simulink model "DvrSimKeybdGD_cs_old"  (R2016a)
settings: Solver=ode5  SolverMode=SingleTasking  StartTime=0.0  StopTime=inf  FixedStep=1/1000  RelTol=1e-3
PreLoadFcn:
  | mbxruntime.callbacks.PreLoadFcn(bdroot);
PostLoadFcn:
  | mbxruntime.callbacks.PostLoadFcn(bdroot);
InitFcn:
  | mbxruntime.callbacks.InitFcn(bdroot);
StartFcn:
  | mbxruntime.callbacks.StartFcn(bdroot);
StopFcn:
  | mbxruntime.callbacks.StopFcn(bdroot);
model workspace (MAT data in the model file):
  mbox_table : struct (value not decoded)
  model_closed = 0
  sim_status = 0
undefined symbols (not defined in the file or in its folder): BMotor1, BMotor2, BrkDelayTime, DControlB, Delay1, Delay2, DiscIntNeverNeededParam, IControlB, JMotor1, JMotor2, PControlB, PreScanCarSimLoadFcn, ratioGearF, ratioGearR, TorqDelayTime, Tstep
undefined symbols (not defined in the file): SteeringColumn, SteeringWheel, WheelL0, WheelL1, WheelR0, WheelR1
libraries: PreScanSimulinkLibrary x35, simulink_extras x26, simulink x26, MyLib x3, Solver_SF x2, pil_lib x1, PreScanUsefulBlocks x1
(part 3 of 12)

== system DvrSimKeybdGD_cs_old/Audi_A8_Sedan_1/Trajectories ==
  Constant1 : Constant  Value=30
  Constant2 : Constant  Value=50
  Discrete-Time Integrator : DiscreteIntegrator  ExternalReset=rising  InitialConditionSource=external  SampleTime=1/20  ICPrevOutput=DiscIntNeverNeededParam  ICPrevScaledInput=DiscIntNeverNeededParam
  ElapsedTrack1 : Subsystem  Tag=ElapsedTrack  mask(PreScan Demux Block:){Filename='Trajectory_2_Path.mat', InitRoll=0, InitPitch=0}
      mask prompts: Filename "Name path-file"; InitRoll "Initial Roll angle (deg):"; InitPitch "Initial Pitch angle (deg):"
      mask init:
      | route=load(['trajectories/',Filename]);
      | 
      | s=route.path(1,:);
      | x=route.path(2,:);
      | y=route.path(3,:);
      | z=route.path(4,:);
      | roll=route.path(5,:);
      | pitch=route.path(6,:);
      | yaw=route.path(7,:);
      settings: DeleteFcn=PreScanBlockDeleteFcn;
  End of Track is reached : Subsystem  Tag=ElapsedTrack  mask(PreScan Demux Block:){Filename='Trajectory_2_Path.mat'}
      mask prompts: Filename "Name path-file"
      mask init:
      | route=load(['trajectories/',Filename]);
      | 
      | s=route.path(1,:);
      | x=route.path(2,:);
      | y=route.path(3,:);
      | yaw=route.path(4,:);
      settings: DeleteFcn=PreScanBlockDeleteFcn;
  Gain : Gain  Gain=1/3.6
  Integrator1 : DiscreteIntegrator  Tag=TrajIntegrator  InitialConditionSetting=State (most efficient)  SampleTime=50/1000  ICPrevOutput=DiscIntNeverNeededParam  ICPrevScaledInput=DiscIntNeverNeededParam
  Memory1 : Memory
  Product : Product  RndMeth=Zero
  Selector1 : Constant  Tag=TrajSubSelector  Value=2
  Step : Step  Before=1  After=0  SampleTime=0
  Terminator_1 : Terminator
  Traj2State1 : Subsystem  Tag=Traj2State  mask(PreScan Demux Block:){}
      settings: DeleteFcn=PreScanBlockDeleteFcn;
  TrajCoGOffset : Subsystem  Tag=TrajCoGOffset  mask(Trajectory CoG Offset block){CoGOffsetZ=0.55, InitRoll=0, InitPitch=0}
      mask prompts: CoGOffsetZ "Z-component of CoG Offset [m]:"; InitRoll "Initial Roll angle [deg]:"; InitPitch "Initial Pitch angle [deg]:"
      mask help: A trajectory follows the surface of the road. However the position of a actor is based on the actor's Center of Gravity, which is typically above the road. This block converts from the trajectory along the road surface to the trajectory of the actor's CoG by realigning the z-component of the CoG offset to be normal to the road.
      settings: DeleteFcn=PreScanBlockDeleteFcn;
  TrajSwitch1 : MultiPortSwitch  Tag=TrajSubSwitch  Inputs=2
  Trajectory_2 : Subsystem  Tag=Trajectory  mask(PreScan Source Block: Trajectory){FileName='Trajectory_2.mat', TimeStep=50/1000}
      mask prompts: TimeStep "Time Step [s]"
      mask help:
      | The Trajectory block contains the trajectories defined in the PreScan Experiment Editor. The output of the trajectory block is the (vehicle) State.
      |
      | For more information, please click Help.
      mask init:
      | EXPROOT=pwd;  % TODO better construction for locating base experiment
      | 
      | trajfilename = fullfile(EXPROOT,'Trajectories',FileName);
      | load(trajfilename);
      | trajectory=trajectory';
      | 
      | traj.time=trajectory(:,1);%[];
      | traj.signals.values=trajectory(:,2:19);
      | traj.dimensions=18;
      | traj.label='';
      | 
      | SampleTime=traj.time(2)-traj.time(1);
      settings: DeleteFcn=PreScanBlockDeleteFcn;
      mask Help: eval('openHelp(312)')
      mask Display: fprintf(FileName)
  Trajectory_2_Offset : Constant  Tag=TrajectoryOffset  Value="[0  0  0  0  0  0]"
  Velocity1 : Constant  Tag=TrajVelocity  Value=15
  State : Outport  Tag=TrajOutport
  wires:
  Constant2/1 -> Product/1
  Product/1 -> Discrete-Time Integrator/3
  Discrete-Time Integrator/1 -> ElapsedTrack1/2(s), Memory1/1
  Memory1/1 -> End of Track is reached/1(s)
  End of Track is reached/1(end_reached) -> Discrete-Time Integrator/2
  Gain/1 -> Discrete-Time Integrator/1
  Constant1/1 -> Gain/1
  Step/1 -> Product/2
  Integrator1/1 -> Terminator_1/1
  Trajectory_2/1(trajectory) -> Traj2State1/1(Traj Org)
  Trajectory_2_Offset/1 -> Traj2State1/2(Offset), ElapsedTrack1/1(Offset)
  Velocity1/1 -> Integrator1/1
  Selector1/1 -> TrajSwitch1/1
  Traj2State1/1(state) -> TrajSwitch1/2
  ElapsedTrack1/1(state) -> TrajSwitch1/3
  TrajCoGOffset/1(State Out) -> State/1
  TrajSwitch1/1 -> TrajCoGOffset/1(State In)

== system DvrSimKeybdGD_cs_old/BMW_X5_SUV_1/SELF_Demux ==
  SELF : Inport  OutDataTypeStr=Bus: PRESCAN_SELFSENSORDATA
  Bus Selector : BusSelector  OutputSignals=PositionX,PositionY,PositionZ,OrientationRoll,OrientationPitch,OrientationYaw,Velocity,Yaw_rate,Lat,Long,Alt
  Demux2 : Demux  Outputs=3
  Gain : Gain  Gain=180/pi
  Gain1 : Gain  Gain=180/pi
  Vector Concatenate1 : Concatenate  NumInputs=3
  compas converter : Subsystem
  x [m] : Outport
  y [m] : Outport  Port=2
  z [m] : Outport  Port=3
  rotx [deg] : Outport  Port=4
  roty [deg] : Outport  Port=5
  rotz [deg] : Outport  Port=6
  GPS lat [deg] : Outport  Port=7
  GPS long [deg] : Outport  Port=8
  GPS alt [m] : Outport  Port=9
  velocity [m/s] : Outport  Port=10
  heading [deg] : Outport  Port=11
  yaw rate [deg/s] : Outport  Port=12
  wires:
  Bus Selector/11 -> GPS alt [m]/1  "<Alt>"
  Bus Selector/10 -> GPS long [deg]/1  "<Long>"
  Bus Selector/9 -> GPS lat [deg]/1  "<Lat>"
  Bus Selector/8 -> Gain1/1  "<Yaw_rate>"
  Bus Selector/7 -> velocity [m/s]/1  "<Velocity>"
  Bus Selector/6 -> compas converter/1(rotz [rad]), Vector Concatenate1/3  "<OrientationYaw>"
  Bus Selector/5 -> Vector Concatenate1/2  "<OrientationPitch>"
  Bus Selector/4 -> Vector Concatenate1/1  "<OrientationRoll>"
  Vector Concatenate1/1 -> Gain/1
  Bus Selector/3 -> z [m]/1  "<PositionZ>"
  Bus Selector/2 -> y [m]/1  "<PositionY>"
  Bus Selector/1 -> x [m]/1  "<PositionX>"
  SELF/1 -> Bus Selector/1
  Gain/1 -> Demux2/1
  Demux2/1 -> rotx [deg]/1
  Demux2/2 -> roty [deg]/1
  Demux2/3 -> rotz [deg]/1
  compas converter/1(heading [deg]) -> heading [deg]/1
  Gain1/1 -> yaw rate [deg/s]/1

== system DvrSimKeybdGD_cs_old/BMW_X5_SUV_1/STATE_BMW_X5_SUV_1 ==
  State : Inport  SampleTime=TimeStep
  Bus Creator : BusCreator  Inputs=15  OutDataTypeStr=Bus: PRESCAN_STATEACTUATORDATA  NonVirtualBus=on
  Demux : Demux  Outputs=15
  iniBODYAngles wrtVEH [rad] : Constant  Value=[Roll0 Pitch0 0]  SampleTime=TimeStep
  iniVEHAngles wrtGLOB [rad] : Constant  Value=[0 0 Yaw0]  SampleTime=TimeStep
  iniVEHposition wrtGLOB [m] : Constant  Value=[x0 y0 z0]  SampleTime=TimeStep
  state2FullState : PreScanSimulinkLibrary/state2FullState  SystemSampleTime=-1
  StateBus : Outport  OutDataTypeStr=Bus: PRESCAN_STATEACTUATORDATA
  wires:
  Bus Creator/1 -> StateBus/1
  State/1 -> state2FullState/1
  state2FullState/1 -> Demux/1
  iniVEHposition wrtGLOB [m]/1 -> state2FullState/2
  iniBODYAngles wrtVEH [rad]/1 -> state2FullState/3
  iniVEHAngles wrtGLOB [rad]/1 -> state2FullState/4
  Demux/1 -> Bus Creator/1  "PositionX"
  Demux/2 -> Bus Creator/2  "PositionY"
  Demux/3 -> Bus Creator/3  "PositionZ"
  Demux/4 -> Bus Creator/4  "VelocityX"
  Demux/5 -> Bus Creator/5  "VelocityY"
  Demux/6 -> Bus Creator/6  "VelocityZ"
  Demux/7 -> Bus Creator/7  "AccelerationX"
  Demux/8 -> Bus Creator/8  "AccelerationY"
  Demux/9 -> Bus Creator/9  "AccelerationZ"
  Demux/10 -> Bus Creator/10  "OrientationRoll"
  Demux/11 -> Bus Creator/11  "OrientationPitch"
  Demux/12 -> Bus Creator/12  "OrientationYaw"
  Demux/13 -> Bus Creator/13  "AngularVelocityRoll"
  Demux/14 -> Bus Creator/14  "AngularVelocityPitch"
  Demux/15 -> Bus Creator/15  "AngularVelocityYaw"

== system DvrSimKeybdGD_cs_old/BMW_X5_SUV_1/Trajectories ==
  Constant1 : Constant  Value=30
  Constant2 : Constant  Value=50
  Discrete-Time Integrator : DiscreteIntegrator  ExternalReset=rising  InitialConditionSource=external  SampleTime=1/20  ICPrevOutput=DiscIntNeverNeededParam  ICPrevScaledInput=DiscIntNeverNeededParam
  ElapsedTrack1 : Subsystem  Tag=ElapsedTrack  mask(PreScan Demux Block:){Filename='Trajectory_4_Path.mat', InitRoll=0, InitPitch=0}
      mask prompts: Filename "Name path-file"; InitRoll "Initial Roll angle (deg):"; InitPitch "Initial Pitch angle (deg):"
      mask init:
      | route=load(['trajectories/',Filename]);
      | 
      | s=route.path(1,:);
      | x=route.path(2,:);
      | y=route.path(3,:);
      | z=route.path(4,:);
      | roll=route.path(5,:);
      | pitch=route.path(6,:);
      | yaw=route.path(7,:);
      settings: DeleteFcn=PreScanBlockDeleteFcn;
  End of Track is reached : Subsystem  Tag=ElapsedTrack  mask(PreScan Demux Block:){Filename='Trajectory_4_Path.mat'}
      mask prompts: Filename "Name path-file"
      mask init:
      | route=load(['trajectories/',Filename]);
      | 
      | s=route.path(1,:);
      | x=route.path(2,:);
      | y=route.path(3,:);
      | yaw=route.path(4,:);
      settings: DeleteFcn=PreScanBlockDeleteFcn;
  Gain : Gain  Gain=1/3.6
  Integrator1 : DiscreteIntegrator  Tag=TrajIntegrator  InitialConditionSetting=State (most efficient)  SampleTime=50/1000  ICPrevOutput=DiscIntNeverNeededParam  ICPrevScaledInput=DiscIntNeverNeededParam
  Memory1 : Memory
  Product : Product  RndMeth=Zero
  Selector1 : Constant  Tag=TrajSubSelector  Value=2
  Step : Step  Before=1  After=0  SampleTime=0
  Terminator_1 : Terminator
  Traj2State1 : Subsystem  Tag=Traj2State  mask(PreScan Demux Block:){}
      settings: DeleteFcn=PreScanBlockDeleteFcn;
  TrajCoGOffset : Subsystem  Tag=TrajCoGOffset  mask(Trajectory CoG Offset block){CoGOffsetZ=0.69, InitRoll=0, InitPitch=0}
      mask prompts: CoGOffsetZ "Z-component of CoG Offset [m]:"; InitRoll "Initial Roll angle [deg]:"; InitPitch "Initial Pitch angle [deg]:"
      mask help: A trajectory follows the surface of the road. However the position of a actor is based on the actor's Center of Gravity, which is typically above the road. This block converts from the trajectory along the road surface to the trajectory of the actor's CoG by realigning the z-component of the CoG offset to be normal to the road.
      settings: DeleteFcn=PreScanBlockDeleteFcn;
  TrajSwitch1 : MultiPortSwitch  Tag=TrajSubSwitch  Inputs=2
  Trajectory_4 : Subsystem  Tag=Trajectory  mask(PreScan Source Block: Trajectory){FileName='Trajectory_4.mat', TimeStep=50/1000}
      mask prompts: TimeStep "Time Step [s]"
      mask help:
      | The Trajectory block contains the trajectories defined in the PreScan Experiment Editor. The output of the trajectory block is the (vehicle) State.
      |
      | For more information, please click Help.
      mask init: same as DvrSimKeybdGD_cs_old/Audi_A8_Sedan_1/Trajectories/Trajectory_2
      settings: DeleteFcn=PreScanBlockDeleteFcn;
      mask Help: eval('openHelp(312)')
      mask Display: fprintf(FileName)
  Trajectory_4_Offset : Constant  Tag=TrajectoryOffset  Value="[0  0  0  0  0  0]"
  Velocity1 : Constant  Tag=TrajVelocity  Value=15
  State : Outport  Tag=TrajOutport
  wires:
  Constant2/1 -> Product/1
  Product/1 -> Discrete-Time Integrator/3
  Discrete-Time Integrator/1 -> ElapsedTrack1/2(s), Memory1/1
  Memory1/1 -> End of Track is reached/1(s)
  End of Track is reached/1(end_reached) -> Discrete-Time Integrator/2
  Gain/1 -> Discrete-Time Integrator/1
  Constant1/1 -> Gain/1
  Step/1 -> Product/2
  Integrator1/1 -> Terminator_1/1
  Trajectory_4/1(trajectory) -> Traj2State1/1(Traj Org)
  Trajectory_4_Offset/1 -> Traj2State1/2(Offset), ElapsedTrack1/1(Offset)
  Velocity1/1 -> Integrator1/1
  Selector1/1 -> TrajSwitch1/1
  Traj2State1/1(state) -> TrajSwitch1/2
  ElapsedTrack1/1(state) -> TrajSwitch1/3
  TrajCoGOffset/1(State Out) -> State/1
  TrajSwitch1/1 -> TrajCoGOffset/1(State In)

== system DvrSimKeybdGD_cs_old/BMW_Z3_Convertible_1/SELF_Demux ==
  SELF : Inport  OutDataTypeStr=Bus: PRESCAN_SELFSENSORDATA
  Bus Selector : BusSelector  OutputSignals=PositionX,PositionY,PositionZ,OrientationRoll,OrientationPitch,OrientationYaw,Velocity,Yaw_rate,Lat,Long,Alt
  Demux2 : Demux  Outputs=3
  Gain : Gain  Gain=180/pi
  Gain1 : Gain  Gain=180/pi
  Vector Concatenate1 : Concatenate  NumInputs=3
  compas converter : Subsystem
  x [m] : Outport
  y [m] : Outport  Port=2
  z [m] : Outport  Port=3
  rotx [deg] : Outport  Port=4
  roty [deg] : Outport  Port=5
  rotz [deg] : Outport  Port=6
  GPS lat [deg] : Outport  Port=7
  GPS long [deg] : Outport  Port=8
  GPS alt [m] : Outport  Port=9
  velocity [m/s] : Outport  Port=10
  heading [deg] : Outport  Port=11
  yaw rate [deg/s] : Outport  Port=12
  wires:
  Bus Selector/11 -> GPS alt [m]/1  "<Alt>"
  Bus Selector/10 -> GPS long [deg]/1  "<Long>"
  Bus Selector/9 -> GPS lat [deg]/1  "<Lat>"
  Bus Selector/8 -> Gain1/1  "<Yaw_rate>"
  Bus Selector/7 -> velocity [m/s]/1  "<Velocity>"
  Bus Selector/6 -> compas converter/1(rotz [rad]), Vector Concatenate1/3  "<OrientationYaw>"
  Bus Selector/5 -> Vector Concatenate1/2  "<OrientationPitch>"
  Bus Selector/4 -> Vector Concatenate1/1  "<OrientationRoll>"
  Vector Concatenate1/1 -> Gain/1
  Bus Selector/3 -> z [m]/1  "<PositionZ>"
  Bus Selector/2 -> y [m]/1  "<PositionY>"
  Bus Selector/1 -> x [m]/1  "<PositionX>"
  SELF/1 -> Bus Selector/1
  Gain/1 -> Demux2/1
  Demux2/1 -> rotx [deg]/1
  Demux2/2 -> roty [deg]/1
  Demux2/3 -> rotz [deg]/1
  compas converter/1(heading [deg]) -> heading [deg]/1
  Gain1/1 -> yaw rate [deg/s]/1

== system DvrSimKeybdGD_cs_old/BMW_Z3_Convertible_1/STATE_BMW_Z3_Convertible_1 ==
  State : Inport  SampleTime=TimeStep
  Bus Creator : BusCreator  Inputs=15  OutDataTypeStr=Bus: PRESCAN_STATEACTUATORDATA  NonVirtualBus=on
  Demux : Demux  Outputs=15
  iniBODYAngles wrtVEH [rad] : Constant  Value=[Roll0 Pitch0 0]  SampleTime=TimeStep
  iniVEHAngles wrtGLOB [rad] : Constant  Value=[0 0 Yaw0]  SampleTime=TimeStep
  iniVEHposition wrtGLOB [m] : Constant  Value=[x0 y0 z0]  SampleTime=TimeStep
  state2FullState : PreScanSimulinkLibrary/state2FullState  SystemSampleTime=-1
  StateBus : Outport  OutDataTypeStr=Bus: PRESCAN_STATEACTUATORDATA
  wires:
  Bus Creator/1 -> StateBus/1
  State/1 -> state2FullState/1
  state2FullState/1 -> Demux/1
  iniVEHposition wrtGLOB [m]/1 -> state2FullState/2
  iniBODYAngles wrtVEH [rad]/1 -> state2FullState/3
  iniVEHAngles wrtGLOB [rad]/1 -> state2FullState/4
  Demux/1 -> Bus Creator/1  "PositionX"
  Demux/2 -> Bus Creator/2  "PositionY"
  Demux/3 -> Bus Creator/3  "PositionZ"
  Demux/4 -> Bus Creator/4  "VelocityX"
  Demux/5 -> Bus Creator/5  "VelocityY"
  Demux/6 -> Bus Creator/6  "VelocityZ"
  Demux/7 -> Bus Creator/7  "AccelerationX"
  Demux/8 -> Bus Creator/8  "AccelerationY"
  Demux/9 -> Bus Creator/9  "AccelerationZ"
  Demux/10 -> Bus Creator/10  "OrientationRoll"
  Demux/11 -> Bus Creator/11  "OrientationPitch"
  Demux/12 -> Bus Creator/12  "OrientationYaw"
  Demux/13 -> Bus Creator/13  "AngularVelocityRoll"
  Demux/14 -> Bus Creator/14  "AngularVelocityPitch"
  Demux/15 -> Bus Creator/15  "AngularVelocityYaw"

== system DvrSimKeybdGD_cs_old/BMW_Z3_Convertible_1/Trajectories ==
  Constant1 : Constant  Value=60
  Constant2 : Constant  Value=200
  Discrete-Time Integrator : DiscreteIntegrator  ExternalReset=rising  InitialConditionSource=external  SampleTime=1/20  ICPrevOutput=DiscIntNeverNeededParam  ICPrevScaledInput=DiscIntNeverNeededParam
  ElapsedTrack1 : Subsystem  Tag=ElapsedTrack  mask(PreScan Demux Block:){Filename='Trajectory_1_Path.mat', InitRoll=0, InitPitch=0}
      mask prompts: Filename "Name path-file"; InitRoll "Initial Roll angle (deg):"; InitPitch "Initial Pitch angle (deg):"
      mask init:
      | route=load(['trajectories/',Filename]);
      | 
      | s=route.path(1,:);
      | x=route.path(2,:);
      | y=route.path(3,:);
      | z=route.path(4,:);
      | roll=route.path(5,:);
      | pitch=route.path(6,:);
      | yaw=route.path(7,:);
      settings: DeleteFcn=PreScanBlockDeleteFcn;
  End of Track is reached : Subsystem  Tag=ElapsedTrack  mask(PreScan Demux Block:){Filename='Trajectory_1_Path.mat'}
      mask prompts: Filename "Name path-file"
      mask init:
      | route=load(['trajectories/',Filename]);
      | 
      | s=route.path(1,:);
      | x=route.path(2,:);
      | y=route.path(3,:);
      | yaw=route.path(4,:);
      settings: DeleteFcn=PreScanBlockDeleteFcn;
  Gain : Gain  Gain=1/3.6
  Integrator1 : DiscreteIntegrator  Tag=TrajIntegrator  InitialConditionSetting=State (most efficient)  SampleTime=50/1000  ICPrevOutput=DiscIntNeverNeededParam  ICPrevScaledInput=DiscIntNeverNeededParam
  Memory1 : Memory
  Product : Product  RndMeth=Zero
  Selector1 : Constant  Tag=TrajSubSelector  Value=2
  Step : Step  Before=1  After=0  SampleTime=0
  Terminator_1 : Terminator
  Traj2State1 : Subsystem  Tag=Traj2State  mask(PreScan Demux Block:){}
      settings: DeleteFcn=PreScanBlockDeleteFcn;
  TrajCoGOffset : Subsystem  Tag=TrajCoGOffset  mask(Trajectory CoG Offset block){CoGOffsetZ=0.4784, InitRoll=0, InitPitch=0}
      mask prompts: CoGOffsetZ "Z-component of CoG Offset [m]:"; InitRoll "Initial Roll angle [deg]:"; InitPitch "Initial Pitch angle [deg]:"
      mask help: A trajectory follows the surface of the road. However the position of a actor is based on the actor's Center of Gravity, which is typically above the road. This block converts from the trajectory along the road surface to the trajectory of the actor's CoG by realigning the z-component of the CoG offset to be normal to the road.
      settings: DeleteFcn=PreScanBlockDeleteFcn;
  TrajSwitch1 : MultiPortSwitch  Tag=TrajSubSwitch  Inputs=2
  Trajectory_1 : Subsystem  Tag=Trajectory  mask(PreScan Source Block: Trajectory){FileName='Trajectory_1.mat', TimeStep=50/1000}
      mask prompts: TimeStep "Time Step [s]"
      mask help:
      | The Trajectory block contains the trajectories defined in the PreScan Experiment Editor. The output of the trajectory block is the (vehicle) State.
      |
      | For more information, please click Help.
      mask init: same as DvrSimKeybdGD_cs_old/Audi_A8_Sedan_1/Trajectories/Trajectory_2
      settings: DeleteFcn=PreScanBlockDeleteFcn;
      mask Help: eval('openHelp(312)')
      mask Display: fprintf(FileName)
  Trajectory_1_Offset : Constant  Tag=TrajectoryOffset  Value="[0  0  0  0  0  0]"
  Velocity1 : Constant  Tag=TrajVelocity  Value=15
  State : Outport  Tag=TrajOutport
  wires:
  Constant2/1 -> Product/1
  Product/1 -> Discrete-Time Integrator/3
  Discrete-Time Integrator/1 -> ElapsedTrack1/2(s), Memory1/1
  Memory1/1 -> End of Track is reached/1(s)
  End of Track is reached/1(end_reached) -> Discrete-Time Integrator/2
  Gain/1 -> Discrete-Time Integrator/1
  Constant1/1 -> Gain/1
  Step/1 -> Product/2
  Integrator1/1 -> Terminator_1/1
  Trajectory_1/1(trajectory) -> Traj2State1/1(Traj Org)
  Trajectory_1_Offset/1 -> Traj2State1/2(Offset), ElapsedTrack1/1(Offset)
  Velocity1/1 -> Integrator1/1
  Selector1/1 -> TrajSwitch1/1
  Traj2State1/1(state) -> TrajSwitch1/2
  ElapsedTrack1/1(state) -> TrajSwitch1/3
  TrajCoGOffset/1(State Out) -> State/1
  TrajSwitch1/1 -> TrajCoGOffset/1(State In)

== system DvrSimKeybdGD_cs_old/Ford_Fiesta_Hatchback_1/SELF_Demux ==
  SELF : Inport  OutDataTypeStr=Bus: PRESCAN_SELFSENSORDATA
  Bus Selector : BusSelector  OutputSignals=PositionX,PositionY,PositionZ,OrientationRoll,OrientationPitch,OrientationYaw,Velocity,Yaw_rate,Lat,Long,Alt
  Demux2 : Demux  Outputs=3
  Gain : Gain  Gain=180/pi
  Gain1 : Gain  Gain=180/pi
  Vector Concatenate1 : Concatenate  NumInputs=3
  compas converter : Subsystem
  x [m] : Outport
  y [m] : Outport  Port=2
  z [m] : Outport  Port=3
  rotx [deg] : Outport  Port=4
  roty [deg] : Outport  Port=5
  rotz [deg] : Outport  Port=6
  GPS lat [deg] : Outport  Port=7
  GPS long [deg] : Outport  Port=8
  GPS alt [m] : Outport  Port=9
  velocity [m/s] : Outport  Port=10
  heading [deg] : Outport  Port=11
  yaw rate [deg/s] : Outport  Port=12
  wires:
  Bus Selector/11 -> GPS alt [m]/1  "<Alt>"
  Bus Selector/10 -> GPS long [deg]/1  "<Long>"
  Bus Selector/9 -> GPS lat [deg]/1  "<Lat>"
  Bus Selector/8 -> Gain1/1  "<Yaw_rate>"
  Bus Selector/7 -> velocity [m/s]/1  "<Velocity>"
  Bus Selector/6 -> compas converter/1(rotz [rad]), Vector Concatenate1/3  "<OrientationYaw>"
  Bus Selector/5 -> Vector Concatenate1/2  "<OrientationPitch>"
  Bus Selector/4 -> Vector Concatenate1/1  "<OrientationRoll>"
  Vector Concatenate1/1 -> Gain/1
  Bus Selector/3 -> z [m]/1  "<PositionZ>"
  Bus Selector/2 -> y [m]/1  "<PositionY>"
  Bus Selector/1 -> x [m]/1  "<PositionX>"
  SELF/1 -> Bus Selector/1
  Gain/1 -> Demux2/1
  Demux2/1 -> rotx [deg]/1
  Demux2/2 -> roty [deg]/1
  Demux2/3 -> rotz [deg]/1
  compas converter/1(heading [deg]) -> heading [deg]/1
  Gain1/1 -> yaw rate [deg/s]/1

== system DvrSimKeybdGD_cs_old/Ford_Fiesta_Hatchback_1/STATE_Ford_Fiesta_Hatchback_1 ==
  State : Inport  SampleTime=TimeStep
  Bus Creator : BusCreator  Inputs=15  OutDataTypeStr=Bus: PRESCAN_STATEACTUATORDATA  NonVirtualBus=on
  Demux : Demux  Outputs=15
  iniBODYAngles wrtVEH [rad] : Constant  Value=[Roll0 Pitch0 0]  SampleTime=TimeStep
  iniVEHAngles wrtGLOB [rad] : Constant  Value=[0 0 Yaw0]  SampleTime=TimeStep
  iniVEHposition wrtGLOB [m] : Constant  Value=[x0 y0 z0]  SampleTime=TimeStep
  state2FullState : PreScanSimulinkLibrary/state2FullState  SystemSampleTime=-1
  StateBus : Outport  OutDataTypeStr=Bus: PRESCAN_STATEACTUATORDATA
  wires:
  Bus Creator/1 -> StateBus/1
  State/1 -> state2FullState/1
  state2FullState/1 -> Demux/1
  iniVEHposition wrtGLOB [m]/1 -> state2FullState/2
  iniBODYAngles wrtVEH [rad]/1 -> state2FullState/3
  iniVEHAngles wrtGLOB [rad]/1 -> state2FullState/4
  Demux/1 -> Bus Creator/1  "PositionX"
  Demux/2 -> Bus Creator/2  "PositionY"
  Demux/3 -> Bus Creator/3  "PositionZ"
  Demux/4 -> Bus Creator/4  "VelocityX"
  Demux/5 -> Bus Creator/5  "VelocityY"
  Demux/6 -> Bus Creator/6  "VelocityZ"
  Demux/7 -> Bus Creator/7  "AccelerationX"
  Demux/8 -> Bus Creator/8  "AccelerationY"
  Demux/9 -> Bus Creator/9  "AccelerationZ"
  Demux/10 -> Bus Creator/10  "OrientationRoll"
  Demux/11 -> Bus Creator/11  "OrientationPitch"
  Demux/12 -> Bus Creator/12  "OrientationYaw"
  Demux/13 -> Bus Creator/13  "AngularVelocityRoll"
  Demux/14 -> Bus Creator/14  "AngularVelocityPitch"
  Demux/15 -> Bus Creator/15  "AngularVelocityYaw"

== system DvrSimKeybdGD_cs_old/Ford_Fiesta_Hatchback_1/Trajectories ==
  Constant1 : Constant  Value=60
  Constant2 : Constant  Value=200
  Discrete-Time Integrator : DiscreteIntegrator  ExternalReset=rising  InitialConditionSource=external  SampleTime=1/20  ICPrevOutput=DiscIntNeverNeededParam  ICPrevScaledInput=DiscIntNeverNeededParam
  ElapsedTrack1 : Subsystem  Tag=ElapsedTrack  mask(PreScan Demux Block:){Filename='Trajectory_3_Path.mat', InitRoll=0, InitPitch=0}
      mask prompts: Filename "Name path-file"; InitRoll "Initial Roll angle (deg):"; InitPitch "Initial Pitch angle (deg):"
      mask init:
      | route=load(['trajectories/',Filename]);
      | 
      | s=route.path(1,:);
      | x=route.path(2,:);
      | y=route.path(3,:);
      | z=route.path(4,:);
      | roll=route.path(5,:);
      | pitch=route.path(6,:);
      | yaw=route.path(7,:);
      settings: DeleteFcn=PreScanBlockDeleteFcn;
  End of Track is reached : Subsystem  Tag=ElapsedTrack  mask(PreScan Demux Block:){Filename='Trajectory_3_Path.mat'}
      mask prompts: Filename "Name path-file"
      mask init:
      | route=load(['trajectories/',Filename]);
      | 
      | s=route.path(1,:);
      | x=route.path(2,:);
      | y=route.path(3,:);
      | yaw=route.path(4,:);
      settings: DeleteFcn=PreScanBlockDeleteFcn;
  Gain : Gain  Gain=1/3.6
  Integrator1 : DiscreteIntegrator  Tag=TrajIntegrator  InitialConditionSetting=State (most efficient)  SampleTime=50/1000  ICPrevOutput=DiscIntNeverNeededParam  ICPrevScaledInput=DiscIntNeverNeededParam
  Memory1 : Memory
  Product : Product  RndMeth=Zero
  Selector1 : Constant  Tag=TrajSubSelector  Value=2
  Step : Step  Before=1  After=0  SampleTime=0
  Terminator_1 : Terminator
  Traj2State1 : Subsystem  Tag=Traj2State  mask(PreScan Demux Block:){}
      settings: DeleteFcn=PreScanBlockDeleteFcn;
  TrajCoGOffset : Subsystem  Tag=TrajCoGOffset  mask(Trajectory CoG Offset block){CoGOffsetZ=0.53, InitRoll=0, InitPitch=0}
      mask prompts: CoGOffsetZ "Z-component of CoG Offset [m]:"; InitRoll "Initial Roll angle [deg]:"; InitPitch "Initial Pitch angle [deg]:"
      mask help: A trajectory follows the surface of the road. However the position of a actor is based on the actor's Center of Gravity, which is typically above the road. This block converts from the trajectory along the road surface to the trajectory of the actor's CoG by realigning the z-component of the CoG offset to be normal to the road.
      settings: DeleteFcn=PreScanBlockDeleteFcn;
  TrajSwitch1 : MultiPortSwitch  Tag=TrajSubSwitch  Inputs=2
  Trajectory_3 : Subsystem  Tag=Trajectory  mask(PreScan Source Block: Trajectory){FileName='Trajectory_3.mat', TimeStep=50/1000}
      mask prompts: TimeStep "Time Step [s]"
      mask help:
      | The Trajectory block contains the trajectories defined in the PreScan Experiment Editor. The output of the trajectory block is the (vehicle) State.
      |
      | For more information, please click Help.
      mask init: same as DvrSimKeybdGD_cs_old/Audi_A8_Sedan_1/Trajectories/Trajectory_2
      settings: DeleteFcn=PreScanBlockDeleteFcn;
      mask Help: eval('openHelp(312)')
      mask Display: fprintf(FileName)
  Trajectory_3_Offset : Constant  Tag=TrajectoryOffset  Value="[0  0  0  0  0  0]"
  Velocity1 : Constant  Tag=TrajVelocity  Value=15
  State : Outport  Tag=TrajOutport
  wires:
  Constant2/1 -> Product/1
  Product/1 -> Discrete-Time Integrator/3
  Discrete-Time Integrator/1 -> Memory1/1, ElapsedTrack1/2(s)
  Memory1/1 -> End of Track is reached/1(s)
  End of Track is reached/1(end_reached) -> Discrete-Time Integrator/2
  Gain/1 -> Discrete-Time Integrator/1
  Constant1/1 -> Gain/1
  Step/1 -> Product/2
  Integrator1/1 -> Terminator_1/1
  Trajectory_3/1(trajectory) -> Traj2State1/1(Traj Org)
  Trajectory_3_Offset/1 -> Traj2State1/2(Offset), ElapsedTrack1/1(Offset)
  Velocity1/1 -> Integrator1/1
  Selector1/1 -> TrajSwitch1/1
  Traj2State1/1(state) -> TrajSwitch1/2
  ElapsedTrack1/1(state) -> TrajSwitch1/3
  TrajCoGOffset/1(State Out) -> State/1
  TrajSwitch1/1 -> TrajCoGOffset/1(State In)

== system DvrSimKeybdGD_cs_old/Roewe_550_S_Sedan_1/AIR_1_Demux ==
  AIR : Inport
  Activate_Switch : Subsystem
      mask Display: text(5,10,'')
  Bus Selector : BusSelector  OutputSignals=DATA.Range,DATA.Azimuth,DATA.Elevation,DATA.ID,DATA.Velocity,DATA.Heading
  Data Type Conversion : DataTypeConversion  OutDataTypeStr=double
  For Iterator : ForIterator  ResetStates=reset  IterationLimit=detectableObjects
  Selector : Selector  InputPortWidth=detectableObjects  IndexOptions=Index vector (port)  Indices=[1 3]  OutputSizes=1
  Signal2ArrayOfSignals1 : Subsystem  mask{VECTORLENGTH=detectableObjects}
      mask prompts: VECTORLENGTH "Length of vector"
  Signal2ArrayOfSignals2 : Subsystem  mask{VECTORLENGTH=detectableObjects}
      mask prompts: VECTORLENGTH "Length of vector"
  Signal2ArrayOfSignals3 : Subsystem  mask{VECTORLENGTH=detectableObjects}
      mask prompts: VECTORLENGTH "Length of vector"
  Signal2ArrayOfSignals4 : Subsystem  mask{VECTORLENGTH=detectableObjects}
      mask prompts: VECTORLENGTH "Length of vector"
  Signal2ArrayOfSignals5 : Subsystem  mask{VECTORLENGTH=detectableObjects}
      mask prompts: VECTORLENGTH "Length of vector"
  Signal2ArrayOfSignals6 : Subsystem  mask{VECTORLENGTH=detectableObjects}
      mask prompts: VECTORLENGTH "Length of vector"
  Range [m] : Outport
  Azimuth [deg] : Outport  Port=2
  Elevation [deg] : Outport  Port=3
  ID [-] : Outport  Port=4
  Velocity [m/s] : Outport  Port=5
  Heading [deg] : Outport  Port=6
  wires:
  Data Type Conversion/1 -> ID [-]/1
  Bus Selector/6 -> Signal2ArrayOfSignals6/2(Element)  "<Heading>"
  Signal2ArrayOfSignals6/1(ArrayofElements) -> Activate_Switch/2(Heading)
  Bus Selector/5 -> Signal2ArrayOfSignals5/2(Element)  "<Velocity>"
  Signal2ArrayOfSignals5/1(ArrayofElements) -> Velocity [m/s]/1
  Bus Selector/4 -> Signal2ArrayOfSignals4/2(Element)  "<ID>"
  Signal2ArrayOfSignals4/1(ArrayofElements) -> Data Type Conversion/1, Activate_Switch/1(BeamID)
  Bus Selector/3 -> Signal2ArrayOfSignals3/2(Element)  "<Elevation>"
  Signal2ArrayOfSignals3/1(ArrayofElements) -> Elevation [deg]/1
  Bus Selector/2 -> Signal2ArrayOfSignals1/2(Element)  "<Azimuth>"
  Signal2ArrayOfSignals1/1(ArrayofElements) -> Azimuth [deg]/1
  Signal2ArrayOfSignals2/1(ArrayofElements) -> Range [m]/1
  Bus Selector/1 -> Signal2ArrayOfSignals2/2(Element)  "<Range>"
  Selector/1 -> Bus Selector/1
  For Iterator/1 -> Signal2ArrayOfSignals6/1(LoopIndex), Signal2ArrayOfSignals5/1(LoopIndex), Signal2ArrayOfSignals4/1(LoopIndex), Signal2ArrayOfSignals3/1(LoopIndex), Signal2ArrayOfSignals1/1(LoopIndex), Signal2ArrayOfSignals2/1(LoopIndex), Selector/2
  AIR/1 -> Selector/1
  Activate_Switch/1(On/Off) -> Heading [deg]/1

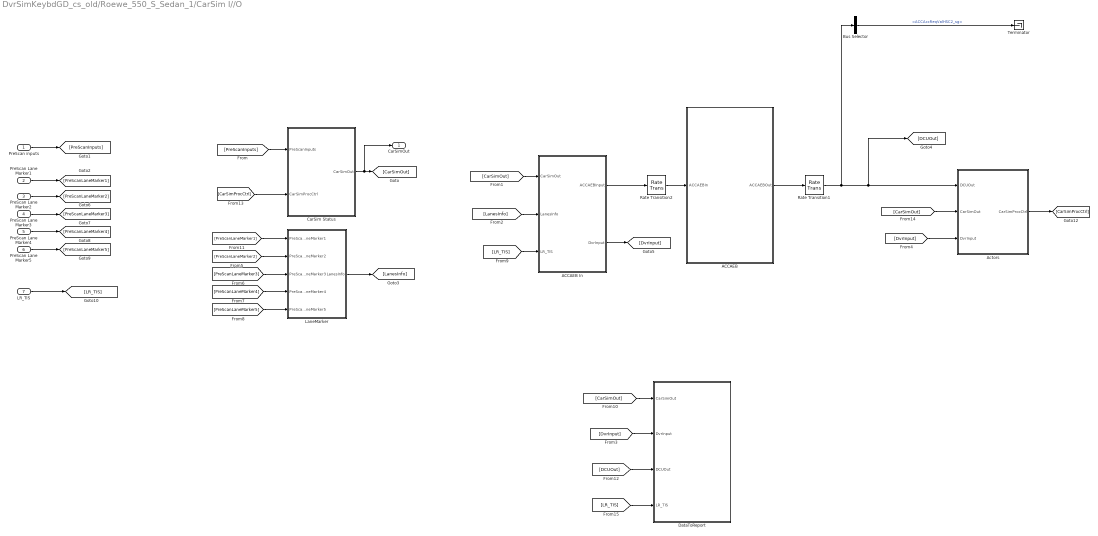
== system DvrSimKeybdGD_cs_old/Roewe_550_S_Sedan_1/CarSim I//O ==
  PreScan inputs : Inport
  PreScan Lane Marker1 : Inport  Port=2
  PreScan Lane Marker2 : Inport  Port=3
  PreScan Lane Marker3 : Inport  Port=4
  PreScan Lane Marker4 : Inport  Port=5
  PreScan Lane Marker5 : Inport  Port=6
  LR_TIS : Inport  Port=7
  ACCAEB : Subsystem  DialogController=pil_create_dialog  LoadFcn=|
      | try
      |    if ~strcmp(rtw.pil.getPILVersion, '6.10 (R2016a)_12')
      |       set_param(gcb, 'DialogController', '');
      |       set_param(gcb, 'DialogControllerArgs', '');
      |    end
      | catch e
      |       set_param(gcb, 'DialogController', '');
      |       set_param(gcb, 'DialogControllerArgs', '');
      | end
      mask help: PIL:pil:XILBlockMaskDesc
      mask Display: disp('SIL S-Function');
  ACCAEB In : Subsystem  TreatAsAtomicUnit=on
  Actors : Subsystem
  Bus Selector : BusSelector  OutputSignals=ACCAccReqValHSC2_sg
  "CarSim Status " : Subsystem  TreatAsAtomicUnit=on
  DataToReport : Subsystem  TreatAsAtomicUnit=on  SystemSampleTime=0.05
  LaneMarker : Subsystem  TreatAsAtomicUnit=on  SystemSampleTime=0.1
  Rate Transition1 : RateTransition  OutPortSampleTime=0.001
  Rate Transition2 : RateTransition  OutPortSampleTime=0.01
  Terminator : Terminator
  CarSimOut : Outport
  wires:
  [PreScanInputs] -> "CarSim Status "/1(PreScanInputs)
  PreScan inputs/1 -> [PreScanInputs]
  PreScan Lane Marker1/1 -> [PreScanLaneMarker1]
  "CarSim Status "/1(CarSimOut) -> CarSimOut/1, [CarSimOut]
  [CarSimOut] -> ACCAEB In/1(CarSimOut)
  [LanesInfo] -> ACCAEB In/2(LanesInfo)
  [LR_TIS] -> ACCAEB In/3(LR_TIS)
  [CarSimProcCtrl] -> "CarSim Status "/2(CarSimProcCtrl)
  PreScan Lane Marker2/1 -> [PreScanLaneMarker2]
  PreScan Lane Marker3/1 -> [PreScanLaneMarker3]
  PreScan Lane Marker4/1 -> [PreScanLaneMarker4]
  PreScan Lane Marker5/1 -> [PreScanLaneMarker5]
  Rate Transition2/1 -> ACCAEB/1(ACCAEBIn)
  ACCAEB In/1(ACCAEBInput) -> Rate Transition2/1
  ACCAEB/1(ACCAEBOut) -> Rate Transition1/1
  Rate Transition1/1 -> Bus Selector/1, [DCUOut], Actors/1(DCUOut)
  [CarSimOut] -> Actors/2(CarSimOut)
  Actors/1(CarSimProcCtrl) -> [CarSimProcCtrl]
  ACCAEB In/2(DvrInput) -> [DvrInput]
  [DvrInput] -> Actors/3(DvrInput)
  LaneMarker/1(LanesInfo) -> [LanesInfo]
  [PreScanLaneMarker4] -> LaneMarker/4(PreScanLaneMarker4)
  [PreScanLaneMarker3] -> LaneMarker/3(PreScanLaneMarker3)
  [PreScanLaneMarker5] -> LaneMarker/5(PreScanLaneMarker5)
  [PreScanLaneMarker2] -> LaneMarker/2(PreScanLaneMarker2)
  [PreScanLaneMarker1] -> LaneMarker/1(PreScanLaneMarker1)
  LR_TIS/1 -> [LR_TIS]
  Bus Selector/1 -> Terminator/1  "<ACCAccReqValHSC2_sg>"
  [DvrInput] -> DataToReport/2(DvrInput)
  [CarSimOut] -> DataToReport/1(CarSimOut)
  [DCUOut] -> DataToReport/3(DCUOut)
  [LR_TIS] -> DataToReport/4(LR_TIS)

== system DvrSimKeybdGD_cs_old/Roewe_550_S_Sedan_1/CarSim_Vehicle ==
  note: For state mode 'Dynamic' positions
      | are not taken into account, as they
      | are computed by integrating velocity.
      | Click annotation for Help.
  Contact_In : Inport
  CarSim S-Function2 : Solver_SF/CarSim S-Function2  Priority=1  VehicleCode=i_i  SIMFILE=simfile.sim
      settings: AttributesFormatString=Vehicle Code: %<VehicleCode>
  CarSim2PreScanSTATE : Subsystem  Tag=CarSim2PreScanSTATE  mask(CarSim2PreScan:){z0=0}
      mask prompts: z0 "PreScan Actor initial COG z-position wrt GLOBAL axis system [m]"
      mask help: This block converts the outputs coming from the CarSim block into consistent PreScan signals.
  CarSim2PreScan_BUS : Subsystem  Tag=CarSim2PreScan_BUS  mask(PreScan block: CarSim to PreScan BUS){TyreRadius=0.44999998807907104, cogZOffset=0}
      mask prompts: TyreRadius "Tyre Radius [m]"; cogZOffset "cog Z offset [m]"
      mask help: CarSim to PreScan BUS selector
      mask Help: eval('openHelp()')
      mask Display: disp('PreScan BUS\nVehicleDynamics')
  CarSim2PreScan_ContactAdapter : Subsystem  Tag=CarSim2PreScan_ContactAdapter  mask{wheelRadius=0.44999998807907104}
      mask prompts: wheelRadius "Wheel radius:"
  MuxState : Subsystem  Tag=mux/State  mask(Empty Dynamics State Block){positioningmode=on, TimeStep=1/1000}
      mask prompts: positioningmode "Positioning Mode"; TimeStep "Auto Assigned: Time Step [s]"
      mask help:
      | Build the state of an actor based on user input.
      | The user can either use positioning mode or dynamics mode.
      | - When using positioning mode the position and orientation of the actor are set directly based on the input. Expected input is relative to the initial position and orientation of the actor. It's also possible to specify the velocity of the actor, though this input isn't used, only passed on.
      | - When using dynamics mode the position input is ignored. Expected input is velocity and orientation. The velocity is relative the current orientation of the actor, while orientation is relative to its initial orientation. The position of the actor is calculated based on the velocity and orientation given.
      settings: DeleteFcn=PreScanBlockDeleteFcn;
  TyreContact To Road Information : Subsystem  Tag=TyreContactToRoadInformation  mask{Roll0=0, Pitch0=0, Yaw0=0}
      mask prompts: Roll0 "Ini roll-angle BODY wrt VEHICLE axis system [deg]"; Pitch0 "Ini pitch-angle BODY wrt VEHICLE axis system [deg]"; Yaw0 "Ini yaw-angle VEHICLE wrt GLOBAL axis system [deg]"
  State : Outport
  State_BUS : Outport  Port=2
  ContactParams : Outport  Port=3
  wires:
  MuxState/1(state) -> State/1, CarSim2PreScan_ContactAdapter/1(State)
  CarSim2PreScanSTATE/1(x [m]) -> MuxState/1(x [m])
  CarSim2PreScanSTATE/2(y [m]) -> MuxState/2(y [m])
  CarSim2PreScanSTATE/3(z [m]) -> MuxState/3(z [m])
  CarSim2PreScanSTATE/4(dx [m/s]) -> MuxState/4(dx [m/s])
  CarSim2PreScanSTATE/5(dy [m/s]) -> MuxState/5(dy [m/s])
  CarSim2PreScanSTATE/6(dz [m/s]) -> MuxState/6(dz [m/s])
  CarSim2PreScanSTATE/7(R [rad]) -> MuxState/7(R [rad])
  CarSim2PreScanSTATE/8(P [rad]) -> MuxState/8(P [rad])
  CarSim2PreScanSTATE/9(Y [rad]) -> MuxState/9(Y [rad])
  CarSim2PreScan_BUS/1(PreScanBUS_VehicleDynamics) -> State_BUS/1, CarSim2PreScan_ContactAdapter/2(State_Bus)
  CarSim S-Function2/1 -> CarSim2PreScanSTATE/1(CarSim_In), CarSim2PreScan_BUS/1(CarSim_In)
  Contact_In/1 -> TyreContact To Road Information/1(TyreInfo_in)
  CarSim2PreScan_ContactAdapter/1(ContactParams) -> ContactParams/1

== system DvrSimKeybdGD_cs_old/Roewe_550_S_Sedan_1/LaneMarkerSensor_1_Data ==
  In1 : Inport
  Bus Creator : BusCreator  Inputs='SliceCount','ScanAtSensor','ScanAtDistance1','ScanAtDistance2','ScanAtDistance3'
  Constant : Constant
  Constant1 : Constant  Value=NUMBEROFSLICES
  Constant2 : Constant  Value=2
  Constant3 : Constant  Value=3
  Constant4 : Constant  Value=4
  Data Type Conversion : DataTypeConversion  OutDataTypeStr=int32
  If{,1..3} (4 alike) : If  NumInputs=2  IfExpression=u1 >= u2  ShowElse=off
  If Action Subsystem1 : Subsystem  TreatAsAtomicUnit=on
  If Action Subsystem2 : Subsystem  TreatAsAtomicUnit=on
  If Action Subsystem3 : Subsystem  TreatAsAtomicUnit=on
  If Action Subsystem4 : Subsystem  TreatAsAtomicUnit=on
  Merge{,1..3} (4 alike) : Merge  InitialOutput=0
  Zero-filled data bus{,1..3} (4 alike) : Constant  Value=0  VectorParams1D=off  OutDataTypeStr=Bus: PRESCAN_LANEMARKER_DATA  SampleTime=TimeStep
  Detection Data : Outport
  wires:
  Data Type Conversion/1 -> Bus Creator/1  "SliceCount"
  In1/1 -> If Action Subsystem2/1(In1), If Action Subsystem4/1(In1), If Action Subsystem3/1(In1), If Action Subsystem1/1(In1)
  Zero-filled data bus3/1 -> Merge3/1
  Zero-filled data bus2/1 -> Merge2/1
  Zero-filled data bus1/1 -> Merge1/1
  Zero-filled data bus/1 -> Merge/1
  Merge3/1 -> Bus Creator/5  "ScanAtDistance3"
  Merge2/1 -> Bus Creator/4  "ScanAtDistance2"
  Merge1/1 -> Bus Creator/3  "ScanAtDistance1"
  If3/1 -> If Action Subsystem4/Action
  If Action Subsystem4/1(Out1) -> Merge3/2
  Constant4/1 -> If3/2, If Action Subsystem4/2(In2)
  If2/1 -> If Action Subsystem3/Action
  If Action Subsystem3/1(Out1) -> Merge2/2
  Constant3/1 -> If Action Subsystem3/2(In2), If2/2
  If1/1 -> If Action Subsystem1/Action
  If Action Subsystem1/1(Out1) -> Merge1/2
  Constant2/1 -> If Action Subsystem1/2(In2), If1/2
  Merge/1 -> Bus Creator/2  "ScanAtSensor"
  Bus Creator/1 -> Detection Data/1
  If/1 -> If Action Subsystem2/Action
  If Action Subsystem2/1(Out1) -> Merge/2
  Constant/1 -> If Action Subsystem2/2(In2), If/2
  Constant1/1 -> Data Type Conversion/1, If3/1, If2/1, If1/1, If/1

== system DvrSimKeybdGD_cs_old/Roewe_550_S_Sedan_1/LaneMarkerSensor_2_Data ==
  In1 : Inport
  Bus Creator : BusCreator  Inputs='SliceCount','ScanAtSensor','ScanAtDistance1','ScanAtDistance2','ScanAtDistance3'
  Constant : Constant
  Constant1 : Constant  Value=NUMBEROFSLICES
  Constant2 : Constant  Value=2
  Constant3 : Constant  Value=3
  Constant4 : Constant  Value=4
  Data Type Conversion : DataTypeConversion  OutDataTypeStr=int32
  If{,1..3} (4 alike) : If  NumInputs=2  IfExpression=u1 >= u2  ShowElse=off
  If Action Subsystem1 : Subsystem  TreatAsAtomicUnit=on
  If Action Subsystem2 : Subsystem  TreatAsAtomicUnit=on
  If Action Subsystem3 : Subsystem  TreatAsAtomicUnit=on
  If Action Subsystem4 : Subsystem  TreatAsAtomicUnit=on
  Merge{,1..3} (4 alike) : Merge  InitialOutput=0
  Zero-filled data bus{,1..3} (4 alike) : Constant  Value=0  VectorParams1D=off  OutDataTypeStr=Bus: PRESCAN_LANEMARKER_DATA  SampleTime=TimeStep
  Detection Data : Outport
  wires:
  Data Type Conversion/1 -> Bus Creator/1  "SliceCount"
  In1/1 -> If Action Subsystem2/1(In1), If Action Subsystem4/1(In1), If Action Subsystem3/1(In1), If Action Subsystem1/1(In1)
  Zero-filled data bus3/1 -> Merge3/1
  Zero-filled data bus2/1 -> Merge2/1
  Zero-filled data bus1/1 -> Merge1/1
  Zero-filled data bus/1 -> Merge/1
  Merge3/1 -> Bus Creator/5  "ScanAtDistance3"
  Merge2/1 -> Bus Creator/4  "ScanAtDistance2"
  Merge1/1 -> Bus Creator/3  "ScanAtDistance1"
  If3/1 -> If Action Subsystem4/Action
  If Action Subsystem4/1(Out1) -> Merge3/2
  Constant4/1 -> If3/2, If Action Subsystem4/2(In2)
  If2/1 -> If Action Subsystem3/Action
  If Action Subsystem3/1(Out1) -> Merge2/2
  Constant3/1 -> If Action Subsystem3/2(In2), If2/2
  If1/1 -> If Action Subsystem1/Action
  If Action Subsystem1/1(Out1) -> Merge1/2
  Constant2/1 -> If Action Subsystem1/2(In2), If1/2
  Merge/1 -> Bus Creator/2  "ScanAtSensor"
  Bus Creator/1 -> Detection Data/1
  If/1 -> If Action Subsystem2/Action
  If Action Subsystem2/1(Out1) -> Merge/2
  Constant/1 -> If Action Subsystem2/2(In2), If/2
  Constant1/1 -> Data Type Conversion/1, If3/1, If2/1, If1/1, If/1

== system DvrSimKeybdGD_cs_old/Roewe_550_S_Sedan_1/LaneMarkerSensor_3_Data ==
  In1 : Inport
  Bus Creator : BusCreator  Inputs='SliceCount','ScanAtSensor','ScanAtDistance1','ScanAtDistance2','ScanAtDistance3'
  Constant : Constant
  Constant1 : Constant  Value=NUMBEROFSLICES
  Constant2 : Constant  Value=2
  Constant3 : Constant  Value=3
  Constant4 : Constant  Value=4
  Data Type Conversion : DataTypeConversion  OutDataTypeStr=int32
  If{,1..3} (4 alike) : If  NumInputs=2  IfExpression=u1 >= u2  ShowElse=off
  If Action Subsystem1 : Subsystem  TreatAsAtomicUnit=on
  If Action Subsystem2 : Subsystem  TreatAsAtomicUnit=on
  If Action Subsystem3 : Subsystem  TreatAsAtomicUnit=on
  If Action Subsystem4 : Subsystem  TreatAsAtomicUnit=on
  Merge{,1..3} (4 alike) : Merge  InitialOutput=0
  Zero-filled data bus{,1..3} (4 alike) : Constant  Value=0  VectorParams1D=off  OutDataTypeStr=Bus: PRESCAN_LANEMARKER_DATA  SampleTime=TimeStep
  Detection Data : Outport
  wires:
  Data Type Conversion/1 -> Bus Creator/1  "SliceCount"
  In1/1 -> If Action Subsystem2/1(In1), If Action Subsystem4/1(In1), If Action Subsystem3/1(In1), If Action Subsystem1/1(In1)
  Zero-filled data bus3/1 -> Merge3/1
  Zero-filled data bus2/1 -> Merge2/1
  Zero-filled data bus1/1 -> Merge1/1
  Zero-filled data bus/1 -> Merge/1
  Merge3/1 -> Bus Creator/5  "ScanAtDistance3"
  Merge2/1 -> Bus Creator/4  "ScanAtDistance2"
  Merge1/1 -> Bus Creator/3  "ScanAtDistance1"
  If3/1 -> If Action Subsystem4/Action
  If Action Subsystem4/1(Out1) -> Merge3/2
  Constant4/1 -> If3/2, If Action Subsystem4/2(In2)
  If2/1 -> If Action Subsystem3/Action
  If Action Subsystem3/1(Out1) -> Merge2/2
  Constant3/1 -> If Action Subsystem3/2(In2), If2/2
  If1/1 -> If Action Subsystem1/Action
  If Action Subsystem1/1(Out1) -> Merge1/2
  Constant2/1 -> If Action Subsystem1/2(In2), If1/2
  Merge/1 -> Bus Creator/2  "ScanAtSensor"
  Bus Creator/1 -> Detection Data/1
  If/1 -> If Action Subsystem2/Action
  If Action Subsystem2/1(Out1) -> Merge/2
  Constant/1 -> If Action Subsystem2/2(In2), If/2
  Constant1/1 -> Data Type Conversion/1, If3/1, If2/1, If1/1, If/1

== system DvrSimKeybdGD_cs_old/Roewe_550_S_Sedan_1/LaneMarkerSensor_4_Data ==
  In1 : Inport
  Bus Creator : BusCreator  Inputs='SliceCount','ScanAtSensor','ScanAtDistance1','ScanAtDistance2','ScanAtDistance3'
  Constant : Constant
  Constant1 : Constant  Value=NUMBEROFSLICES
  Constant2 : Constant  Value=2
  Constant3 : Constant  Value=3
  Constant4 : Constant  Value=4
  Data Type Conversion : DataTypeConversion  OutDataTypeStr=int32
  If{,1..3} (4 alike) : If  NumInputs=2  IfExpression=u1 >= u2  ShowElse=off
  If Action Subsystem1 : Subsystem  TreatAsAtomicUnit=on
  If Action Subsystem2 : Subsystem  TreatAsAtomicUnit=on
  If Action Subsystem3 : Subsystem  TreatAsAtomicUnit=on
  If Action Subsystem4 : Subsystem  TreatAsAtomicUnit=on
  Merge{,1..3} (4 alike) : Merge  InitialOutput=0
  Zero-filled data bus{,1..3} (4 alike) : Constant  Value=0  VectorParams1D=off  OutDataTypeStr=Bus: PRESCAN_LANEMARKER_DATA  SampleTime=TimeStep
  Detection Data : Outport
  wires:
  Data Type Conversion/1 -> Bus Creator/1  "SliceCount"
  In1/1 -> If Action Subsystem2/1(In1), If Action Subsystem4/1(In1), If Action Subsystem3/1(In1), If Action Subsystem1/1(In1)
  Zero-filled data bus3/1 -> Merge3/1
  Zero-filled data bus2/1 -> Merge2/1
  Zero-filled data bus1/1 -> Merge1/1
  Zero-filled data bus/1 -> Merge/1
  Merge3/1 -> Bus Creator/5  "ScanAtDistance3"
  Merge2/1 -> Bus Creator/4  "ScanAtDistance2"
  Merge1/1 -> Bus Creator/3  "ScanAtDistance1"
  If3/1 -> If Action Subsystem4/Action
  If Action Subsystem4/1(Out1) -> Merge3/2
  Constant4/1 -> If3/2, If Action Subsystem4/2(In2)
  If2/1 -> If Action Subsystem3/Action
  If Action Subsystem3/1(Out1) -> Merge2/2
  Constant3/1 -> If Action Subsystem3/2(In2), If2/2
  If1/1 -> If Action Subsystem1/Action
  If Action Subsystem1/1(Out1) -> Merge1/2
  Constant2/1 -> If Action Subsystem1/2(In2), If1/2
  Merge/1 -> Bus Creator/2  "ScanAtSensor"
  Bus Creator/1 -> Detection Data/1
  If/1 -> If Action Subsystem2/Action
  If Action Subsystem2/1(Out1) -> Merge/2
  Constant/1 -> If Action Subsystem2/2(In2), If/2
  Constant1/1 -> Data Type Conversion/1, If3/1, If2/1, If1/1, If/1

== system DvrSimKeybdGD_cs_old/Roewe_550_S_Sedan_1/LaneMarkerSensor_5_Data ==
  In1 : Inport
  Bus Creator : BusCreator  Inputs='SliceCount','ScanAtSensor','ScanAtDistance1','ScanAtDistance2','ScanAtDistance3'
  Constant : Constant
  Constant1 : Constant  Value=NUMBEROFSLICES
  Constant2 : Constant  Value=2
  Constant3 : Constant  Value=3
  Constant4 : Constant  Value=4
  Data Type Conversion : DataTypeConversion  OutDataTypeStr=int32
  If{,1..3} (4 alike) : If  NumInputs=2  IfExpression=u1 >= u2  ShowElse=off
  If Action Subsystem1 : Subsystem  TreatAsAtomicUnit=on
  If Action Subsystem2 : Subsystem  TreatAsAtomicUnit=on
  If Action Subsystem3 : Subsystem  TreatAsAtomicUnit=on
  If Action Subsystem4 : Subsystem  TreatAsAtomicUnit=on
  Merge{,1..3} (4 alike) : Merge  InitialOutput=0
  Zero-filled data bus{,1..3} (4 alike) : Constant  Value=0  VectorParams1D=off  OutDataTypeStr=Bus: PRESCAN_LANEMARKER_DATA  SampleTime=TimeStep
  Detection Data : Outport
  wires:
  Data Type Conversion/1 -> Bus Creator/1  "SliceCount"
  In1/1 -> If Action Subsystem2/1(In1), If Action Subsystem4/1(In1), If Action Subsystem3/1(In1), If Action Subsystem1/1(In1)
  Zero-filled data bus3/1 -> Merge3/1
  Zero-filled data bus2/1 -> Merge2/1
  Zero-filled data bus1/1 -> Merge1/1
  Zero-filled data bus/1 -> Merge/1
  Merge3/1 -> Bus Creator/5  "ScanAtDistance3"
  Merge2/1 -> Bus Creator/4  "ScanAtDistance2"
  Merge1/1 -> Bus Creator/3  "ScanAtDistance1"
  If3/1 -> If Action Subsystem4/Action
  If Action Subsystem4/1(Out1) -> Merge3/2
  Constant4/1 -> If3/2, If Action Subsystem4/2(In2)
  If2/1 -> If Action Subsystem3/Action
  If Action Subsystem3/1(Out1) -> Merge2/2
  Constant3/1 -> If Action Subsystem3/2(In2), If2/2
  If1/1 -> If Action Subsystem1/Action
  If Action Subsystem1/1(Out1) -> Merge1/2
  Constant2/1 -> If Action Subsystem1/2(In2), If1/2
  Merge/1 -> Bus Creator/2  "ScanAtSensor"
  Bus Creator/1 -> Detection Data/1
  If/1 -> If Action Subsystem2/Action
  If Action Subsystem2/1(Out1) -> Merge/2
  Constant/1 -> If Action Subsystem2/2(In2), If/2
  Constant1/1 -> Data Type Conversion/1, If3/1, If2/1, If1/1, If/1
